simulink model "Robot_PID2_model"  (R2016b)
settings: Solver=VariableStepAuto  StartTime=0.0  StopTime=10.0  RelTol=1e-3
values from neighbouring files (symbols this model uses):
  A = [0, 0, 1, 0 ... (first row only)    [Robot_PID.m]    (also in Robot_PID2.m)
  B = [0 ... (first row only)    [Robot_PID.m]    (also in Robot_PID2.m)
  C = [1,0,0,0 ... (first row only)    [Robot_PID.m]    (also in Robot_PID2.m)
  D = [0,0,0,0]'    [Robot_PID.m]    (also in Robot_PID2.m)
  dTheta_0 = 0    [Robot_PID2.m]
  dTheta_y = 0    [Robot_PID2.m]
  Kd1 = 0.00001    (= 1e-05)    [Robot_PID2.m]
  Kd2 = 0.1    [Robot_PID2.m]
  Ki1 = 0.4    [Robot_PID2.m]
  Ki2 = 100    [Robot_PID2.m]
  Kp1 = 0.0001    [Robot_PID2.m]
  Kp2 = 10    [Robot_PID2.m]
  R = 0.04    [Robot_PID.m]    (also in Robot_PID2.m)
libraries: simulink x2
settings Model: Creator=macbookmichal  LastModifiedBy=macbookmichal

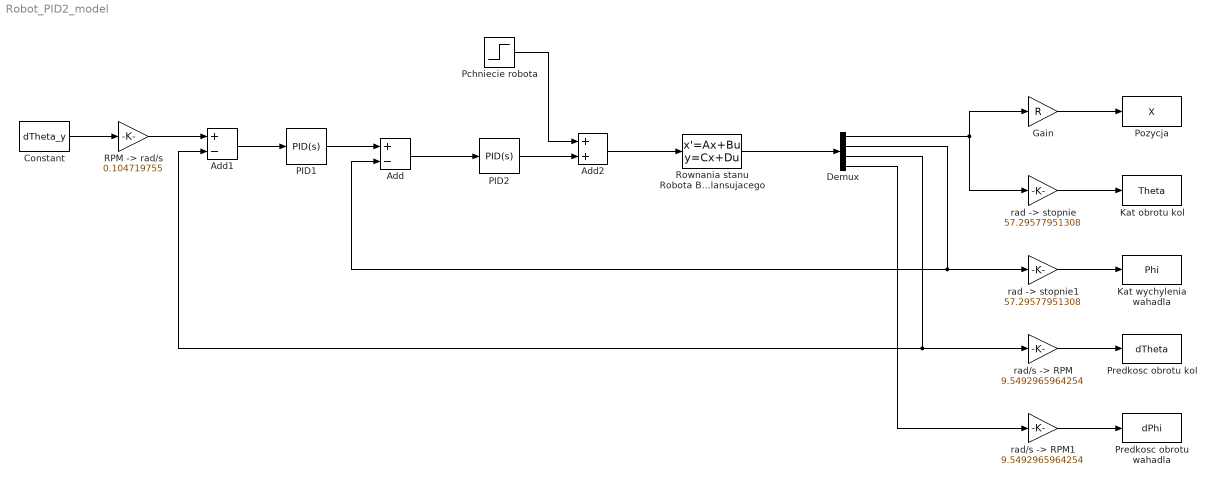
== system Robot_PID2_model ==
  Add : Sum  Inputs=+-
  Add1 : Sum  Inputs=+-
  Add2 : Sum
  Constant : Constant  Value=dTheta_y
  Demux : Demux
  Gain : Gain  Gain=R
  Kat obrotu kol : ToWorkspace  VariableName=Theta  SampleTime=-1
  Kat wychylenia wahadla : ToWorkspace  VariableName=Phi  SampleTime=-1
  PID1 : simulink/Continuous/PID Controller  Controller=PID  TimeDomain=Continuous-time  SampleTime=-1  IntegratorMethod=Forward Euler  FilterMethod=Forward Euler  Form=Parallel  UseFilter=on  ControllerParametersSource=internal  P=Kp1  I=Ki1  D=Kd1  N=100  InitialConditionSource=internal  InitialConditionForIntegrator=0  InitialConditionForFilter=0  ExternalReset=none  LimitOutput=off  UpperSaturationLimit=inf  LowerSaturationLimit=-inf  LinearizeAsGain=on  AntiWindupMode=none  Kb=1  TrackingMode=off  Kt=1  PParamMin=[]  PParamMax=[]  IParamMin=[]  IParamMax=[]  DParamMin=[]  DParamMax=[]  NParamMin=[]  NParamMax=[]  KbParamMin=[]  KbParamMax=[]  KtParamMin=[]  KtParamMax=[]  POutMin=[]  POutMax=[]  IOutMin=[]  IOutMax=[]  DOutMin=[]  DOutMax=[]  NOutMin=[]  NOutMax=[]  KbOutMin=[]  KbOutMax=[]  KtOutMin=[]  KtOutMax=[]  IntegratorOutMin=[]  IntegratorOutMax=[]  FilterOutMin=[]  FilterOutMax=[]  SumOutMin=[]  SumOutMax=[]  SumI1OutMin=[]  SumI1OutMax=[]  SumI2OutMin=[]  SumI2OutMax=[]  SumI3OutMin=[]  SumI3OutMax=[]  SumDOutMin=[]  SumDOutMax=[]  SaturationOutMin=[]  SaturationOutMax=[]  IntegratorContinuousStateAttributes=''  IntegratorStateMustResolveToSignalObject=off  IntegratorRTWStateStorageClass=Auto  FilterContinuousStateAttributes=''  FilterStateMustResolveToSignalObject=off  FilterRTWStateStorageClass=Auto  DifferentiatorICPrevScaledInput=0  DifferentiatorOutMin=[]  DifferentiatorOutMax=[]
  PID2 : simulink/Continuous/PID Controller  Controller=PID  TimeDomain=Continuous-time  SampleTime=-1  IntegratorMethod=Forward Euler  FilterMethod=Forward Euler  Form=Parallel  UseFilter=on  ControllerParametersSource=internal  P=Kp2  I=Ki2  D=Kd2  N=100  InitialConditionSource=internal  InitialConditionForIntegrator=0  InitialConditionForFilter=0  ExternalReset=none  LimitOutput=off  UpperSaturationLimit=inf  LowerSaturationLimit=-inf  LinearizeAsGain=on  AntiWindupMode=none  Kb=1  TrackingMode=off  Kt=1  PParamMin=[]  PParamMax=[]  IParamMin=[]  IParamMax=[]  DParamMin=[]  DParamMax=[]  NParamMin=[]  NParamMax=[]  KbParamMin=[]  KbParamMax=[]  KtParamMin=[]  KtParamMax=[]  POutMin=[]  POutMax=[]  IOutMin=[]  IOutMax=[]  DOutMin=[]  DOutMax=[]  NOutMin=[]  NOutMax=[]  KbOutMin=[]  KbOutMax=[]  KtOutMin=[]  KtOutMax=[]  IntegratorOutMin=[]  IntegratorOutMax=[]  FilterOutMin=[]  FilterOutMax=[]  SumOutMin=[]  SumOutMax=[]  SumI1OutMin=[]  SumI1OutMax=[]  SumI2OutMin=[]  SumI2OutMax=[]  SumI3OutMin=[]  SumI3OutMax=[]  SumDOutMin=[]  SumDOutMax=[]  SaturationOutMin=[]  SaturationOutMax=[]  IntegratorContinuousStateAttributes=''  IntegratorStateMustResolveToSignalObject=off  IntegratorRTWStateStorageClass=Auto  FilterContinuousStateAttributes=''  FilterStateMustResolveToSignalObject=off  FilterRTWStateStorageClass=Auto  DifferentiatorICPrevScaledInput=0  DifferentiatorOutMin=[]  DifferentiatorOutMax=[]
  Pchniecie robota : Step  After=0.25  SampleTime=0
  Pozycja : ToWorkspace  VariableName=X  SampleTime=-1
  Predkosc obrotu kol : ToWorkspace  VariableName=dTheta  SampleTime=-1
  Predkosc obrotu wahadla : ToWorkspace  VariableName=dPhi  SampleTime=-1
  "RPM -> rad/s" : Gain  Gain=0.104719755
  Rownania stanu Robota Balansujacego : StateSpace  A=A  B=B  C=C  D=D  X0=dTheta_0 * 0.01745329251
  "rad -> stopnie" : Gain  Gain=57.29577951308
  "rad -> stopnie1" : Gain  Gain=57.29577951308
  "rad/s -> RPM" : Gain  Gain=9.5492965964254
  "rad/s -> RPM1" : Gain  Gain=9.5492965964254
  wires:
  Add/1 -> PID2/1
  Rownania stanu Robota Balansujacego/1 -> Demux/1
  PID1/1 -> Add/1
  Add1/1 -> PID1/1
  Gain/1 -> Pozycja/1
  Demux/1 -> "rad -> stopnie"/1, Gain/1
  Demux/2 -> Add/2, "rad -> stopnie1"/1
  "rad -> stopnie"/1 -> Kat obrotu kol/1
  "rad -> stopnie1"/1 -> Kat wychylenia wahadla/1
  "rad/s -> RPM"/1 -> Predkosc obrotu kol/1
  "rad/s -> RPM1"/1 -> Predkosc obrotu wahadla/1
  Demux/3 -> "rad/s -> RPM"/1, Add1/2
  Demux/4 -> "rad/s -> RPM1"/1
  Constant/1 -> "RPM -> rad/s"/1
  "RPM -> rad/s"/1 -> Add1/1
  Add2/1 -> Rownania stanu Robota Balansujacego/1
  PID2/1 -> Add2/2
  Pchniecie robota/1 -> Add2/1
